simulink model "model"  (R2023a)
settings: Solver=ode4  StartTime=0.0  StopTime=100  FixedStep=0.01  RelTol=1e-3
values from neighbouring files (symbols this model uses):
  B_p_eq = (g_w^2 * b_m) + (r_p^2 * b_r)    [load_params.m]
  g_w = z2 / z1    [load_params.m]
  J_p_eq = (g_w^2 * j_m) + (r_p^2 * m_r)    [load_params.m]
  k_c = (g_st * I_p) / l_tb    [load_params.m]
  r_p = maskInitContext.MaskWorkspace.get('r_p')    [Mask_Pacejka.m]    (also in load_params.m = c_lk / (2 * pi))
  T_fp_eq = r_p * f_fr    [load_params.m]
undefined symbols (not defined in the file or in its folder): b_c, t_fc
settings Model: Creator=ADMIN  LastModifiedBy=ADMIN

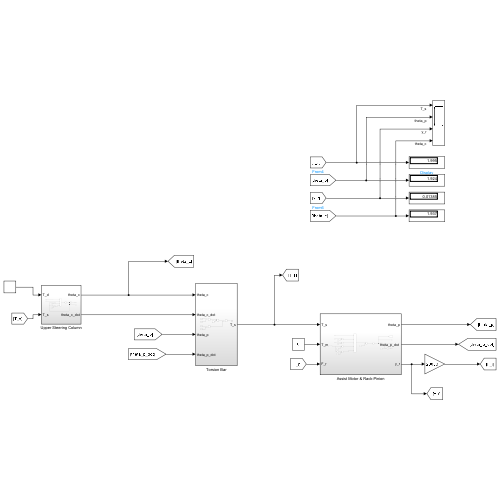
[thumbnail: Simulink's stored preview of the top-level diagram]
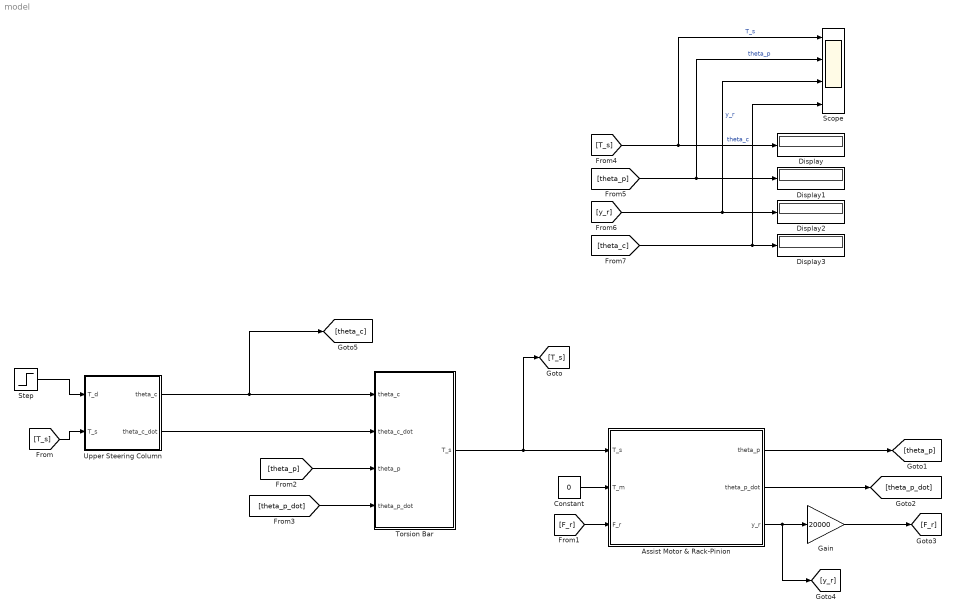
== system model ==
  Assist Motor & Rack-Pinion : Subsystem
  Constant : Constant  Value=0
  Display{,1..3} (4 alike) : Display
  Gain : Gain  Gain=20000
  Scope : Scope  NumInputPorts=4
  Step : Step  After=2  SampleTime=0
  Torsion Bar : Subsystem
  Upper Steering Column : Subsystem
  wires:
  Upper Steering Column/1(theta_c) -> [theta_c], Torsion Bar/1(theta_c)
  Upper Steering Column/2(theta_c_dot) -> Torsion Bar/2(theta_c_dot)
  Step/1 -> Upper Steering Column/1(T_d)
  Torsion Bar/1(T_s) -> [T_s], Assist Motor & Rack-Pinion/1(T_s)
  [T_s] -> Upper Steering Column/2(T_s)
  Assist Motor & Rack-Pinion/1(theta_p) -> [theta_p]
  Assist Motor & Rack-Pinion/2("theta_p_dot ") -> [theta_p_dot]
  Assist Motor & Rack-Pinion/3(y_r) -> [y_r], Gain/1
  Gain/1 -> [F_r]
  [F_r] -> Assist Motor & Rack-Pinion/3(F_r)
  [theta_p] -> Torsion Bar/3(theta_p)
  [theta_p_dot] -> Torsion Bar/4(theta_p_dot)
  Constant/1 -> Assist Motor & Rack-Pinion/2(T_m)
  [T_s] -> Scope/1, Display/1  "T_s"
  [theta_p] -> Scope/2, Display1/1  "theta_p"
  [y_r] -> Scope/3, Display2/1  "y_r"
  [theta_c] -> Scope/4, Display3/1  "theta_c"

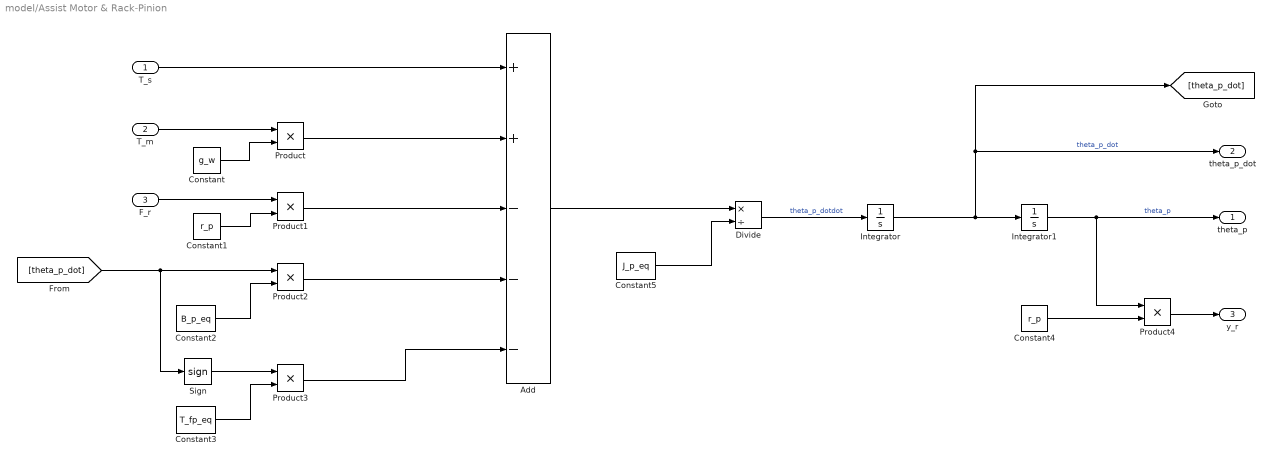
== system model/Assist Motor & Rack-Pinion ==
  T_s : Inport
  T_m : Inport  Port=2
  F_r : Inport  Port=3
  Add : Sum  Inputs=++---
  Constant : Constant  Value=g_w
  Constant1 : Constant  Value=r_p
  Constant2 : Constant  Value=B_p_eq
  Constant3 : Constant  Value=T_fp_eq
  Constant4 : Constant  Value=r_p
  Constant5 : Constant  Value=J_p_eq
  Divide : Product  Inputs=*/
  Integrator : Integrator
  Integrator1 : Integrator
  Product{,1..4} (5 alike) : Product
  Sign : Signum
  theta_p : Outport
  "theta_p_dot " : Outport  Port=2
  y_r : Outport  Port=3
  wires:
  T_m/1 -> Product/1
  Constant/1 -> Product/2
  F_r/1 -> Product1/1
  Constant1/1 -> Product1/2
  Product/1 -> Add/2
  Product1/1 -> Add/3
  T_s/1 -> Add/1
  Add/1 -> Divide/1
  Integrator/1 -> "theta_p_dot "/1, [theta_p_dot], Integrator1/1  "theta_p_dot"
  Integrator1/1 -> Product4/1, theta_p/1  "theta_p"
  Constant2/1 -> Product2/2
  Product2/1 -> Add/4
  [theta_p_dot] -> Sign/1, Product2/1
  Constant3/1 -> Product3/2
  Sign/1 -> Product3/1
  Product3/1 -> Add/5
  Product4/1 -> y_r/1
  Divide/1 -> Integrator/1  "theta_p_dotdot"
  Constant4/1 -> Product4/2
  Constant5/1 -> Divide/2

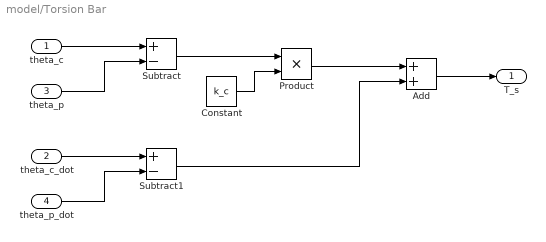
== system model/Torsion Bar ==
  theta_c : Inport
  theta_c_dot : Inport  Port=2
  theta_p : Inport  Port=3
  theta_p_dot : Inport  Port=4
  Add : Sum
  Constant : Constant  Value=k_c
  Product : Product
  Subtract : Sum  Inputs=+-
  Subtract1 : Sum  Inputs=+-
  T_s : Outport
  wires:
  theta_c/1 -> Subtract/1
  theta_p/1 -> Subtract/2
  Subtract/1 -> Product/1
  Constant/1 -> Product/2
  Product/1 -> Add/1
  Add/1 -> T_s/1
  theta_c_dot/1 -> Subtract1/1
  theta_p_dot/1 -> Subtract1/2
  Subtract1/1 -> Add/2

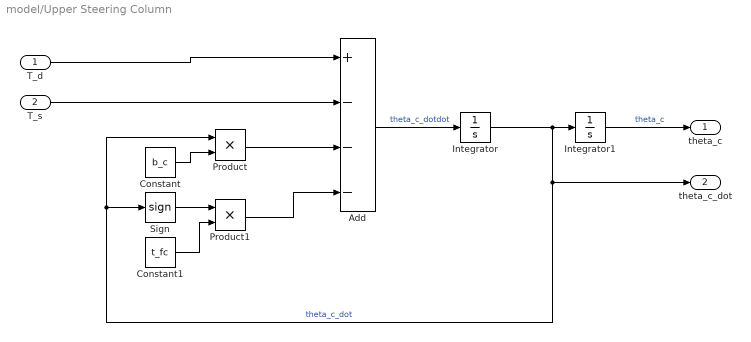
== system model/Upper Steering Column ==
  T_d : Inport
  T_s : Inport  Port=2
  Add : Sum  Inputs=+---
  Constant : Constant  Value=b_c
  Constant1 : Constant  Value=t_fc
  Integrator : Integrator
  Integrator1 : Integrator
  Product : Product
  Product1 : Product
  Sign : Signum
  theta_c : Outport
  theta_c_dot : Outport  Port=2
  wires:
  T_d/1 -> Add/1
  T_s/1 -> Add/2
  Constant/1 -> Product/2
  Product/1 -> Add/3
  Add/1 -> Integrator/1  "theta_c_dotdot"
  Integrator/1 -> Integrator1/1, Product/1, Sign/1, theta_c_dot/1  "theta_c_dot"
  Integrator1/1 -> theta_c/1  "theta_c"
  Constant1/1 -> Product1/2
  Product1/1 -> Add/4
  Sign/1 -> Product1/1
